simulink model "MCP_phase3_LQR"  (R2020a)
settings: Solver=VariableStepAuto  StartTime=0.0  StopTime=400  RelTol=1e-3
values from neighbouring files (symbols this model uses):
  eq_values = zeros(4,1)    [Four_Tank_phase3_LQR.m]
  h1_eq = 11.4    [Four_Tank.m]    (also in Four_Tank_phase3_LQR.m; Four_Tank_phase3_nonlinear.m; MCP_phase3_observers.m)
  h2_eq = 11.6    [Four_Tank.m]    (also in Four_Tank_phase3_LQR.m; Four_Tank_phase3_nonlinear.m; MCP_phase3_observers.m)
  h3_eq = 5.3    [Four_Tank.m]    (also in Four_Tank_phase3_LQR.m; Four_Tank_phase3_nonlinear.m = real(double(answer.h3)); MCP_phase3_observers.m)
  h4_eq = 4    [Four_Tank.m]    (also in Four_Tank_phase3_LQR.m; Four_Tank_phase3_nonlinear.m = real(double(answer.h4)); MCP_phase3_observers.m)
settings Model: Creator=rafiee  LastModifiedBy=Lenovo
settings DataIOCC: ReturnWorkspaceOutputs=off
settings DebuggingCC: ArithmeticOperatorsInVariantConditions=warning
settings SFSimCC: SimUseLocalCustomCode=off  CustomCodeUndefinedFunction=UseInterfaceOnly
settings RTWCC: RTWUseLocalCustomCode=off
settings CodeAppCC: StateflowObjectComments=on

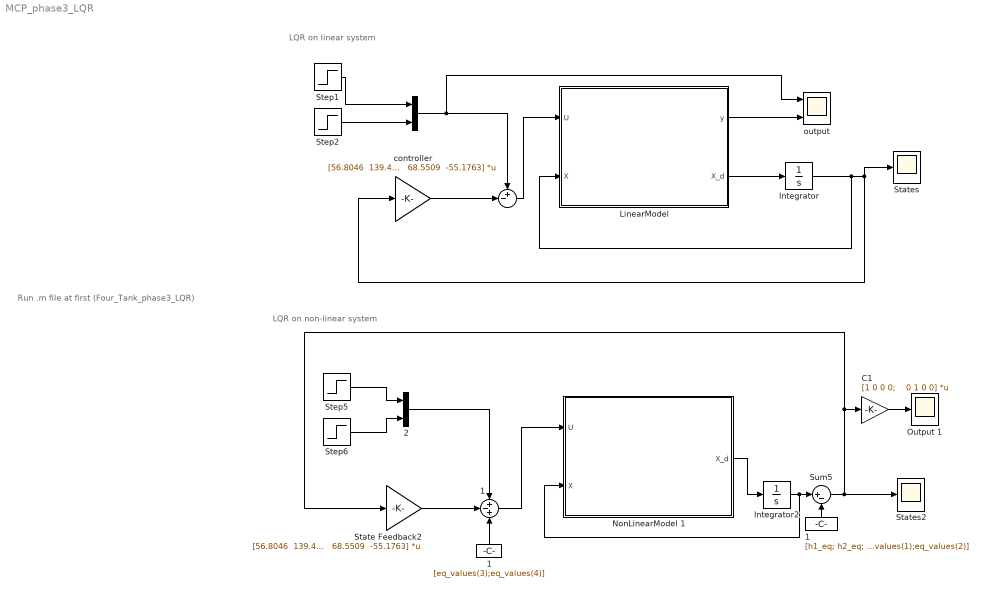
== system MCP_phase3_LQR ==
  note: LQR on linear system
  note: LQR on non-linear system
  note: Run .m file at first (Four_Tank_phase3_LQR)
  " " : Sum  Inputs=+-|
  "   " : Concatenate
  "                             1" : Constant  Value=[h1_eq; h2_eq; eq_values(1);eq_values(2)]
  "                        1" : Constant  Value=[eq_values(3);eq_values(4)]
  "        1" : Sum  Inputs=+-+
  "   2" : Concatenate
  C1 : Gain  Gain=|  Multiplication=Matrix(K*u)
      | [1 0 0 0;
      |    0 1 0 0]
  "Integrator  " : Integrator  InitialCondition=|
      | [0
      | ;0
      | ; -0.1943
      | ; 0.1518]
  Integrator2 : Integrator  InitialCondition=[h1_eq;h2_eq;h3_eq;h4_eq]
  LinearModel : MATLAB Function  TreatAsAtomicUnit=on
  NonLinearModel 1 : MATLAB Function  TreatAsAtomicUnit=on
  Output 1 : Scope
  State Feedback2 : Gain  Gain="[56.8046  139.4053  -70.4297   74.0215;138.5844   98.5390   68.5509  -55.1763]"  Multiplication=Matrix(K*u)
  States : Scope
  States2 : Scope
  Step{1..2,5..6} (4 alike) : Step  SampleTime=0
  Sum5 : Sum  Inputs=|+-
  controller : Gain  Gain="[56.8046  139.4053  -70.4297   74.0215;138.5844   98.5390   68.5509  -55.1763]"  Multiplication=Matrix(K*u)
  output : Scope  NumInputPorts=2
  wires:
  "   "/1 -> " "/1, output/1
  Step2/1 -> "   "/2
  LinearModel/2(X_d) -> "Integrator  "/1
  Step1/1 -> "   "/1
  "Integrator  "/1 -> LinearModel/2(X), States/1, controller/1
  " "/1 -> LinearModel/1(U)
  LinearModel/1(y) -> output/2
  controller/1 -> " "/2
  "                        1"/1 -> "        1"/3
  "                             1"/1 -> Sum5/2
  Step6/1 -> "   2"/2
  "   2"/1 -> "        1"/1
  "        1"/1 -> NonLinearModel 1/1(U)
  C1/1 -> Output 1/1
  Step5/1 -> "   2"/1
  State Feedback2/1 -> "        1"/2
  NonLinearModel 1/1(X_d) -> Integrator2/1
  Integrator2/1 -> Sum5/1, NonLinearModel 1/2(X)
  Sum5/1 -> C1/1, State Feedback2/1, States2/1

== matlab function MCP_phase3_LQR/NonLinearModel 1 ==
  data: U input; X input; X_d output
function X_d   = non_linear_plant(U,X)
Area = [730 730 730 730]; % area of the tanks in cm^2
a = [2.10 2.14 2.2 2.3];  % area of the drain in cm^2
y = [0.3 0.35];           % y(1) = Ratio of flow in tank1 to flow in tank4
                          % y(2) = Ratio of flow in tank2 to flow in tank3                   
k = [7.45 7.30];          % pump proportionality constants in cm^2/s
g = 981;                  % gravitational acceleration in cm/s^2

h1 = X(1);
h2 = X(2);
h3 = X(3);
h4 = X(4);

v1 = U(1);
v2 = U(2);

h1_d = -a(1)/Area(1)*sqrt(2*g*h1)+a(3)/Area(1)*sqrt(2*g*h3)+y(1)*k(1)/Area(1)*v1+0.00137;
h2_d = -a(2)/Area(2)*sqrt(2*g*h2)+a(4)/Area(2)*sqrt(2*g*h4)+y(2)*k(2)/Area(2)*v2+0.00137;
h3_d = -a(3)/Area(3)*sqrt(2*g*h3)+(1 - y(2))*k(2)/Area(3)*v2;
h4_d = -a(4)/Area(4)*sqrt(2*g*h4)+(1 - y(1))*k(1)/Area(4)*v1;

X_d = [h1_d;h2_d;h3_d;h4_d];

== matlab function MCP_phase3_LQR/LinearModel ==
  data: U input; y output; X input; X_d output
function [y,X_d]  = linear_plant(U,X)
% A = [ -0.0189,  0.029,      0, 0.00306,       0,       0;
%        0, -0.029, 0.0065,       0,       0,       0;
%        0,      0, -0.476,       0,       0,       0;
%        0,      0,      0,    -0.5,       0,       0;
%        0,      0, 0.0035,       0, -0.0191,  0.0349;
%        0,      0,      0, 0.00714,       0, -0.0349];
% 
% B =[0,     0;
%    0,     0;
%    0, 0.476;
%    0.5,     0;
%    0,     0;
%    0,     0];
% 
% C = [1.0, 0, 0, 0, 0, 0;
%      0, 0, 0, 0, 1.0, 0];

A = [   -0.0189         0    0.0290         0;
         0   -0.0191         0    0.0349;
         0         0   -0.0290         0;
         0         0         0   -0.0349];
     
B = [ 0.0031         0;
         0    0.0035;
         0    0.0065;
    0.0071         0];
C =[1     0     0     0;
     0     1     0     0];

     
X_d = A * X + B * U; 
y = C*X;
